simulink model "multitapdelay"  (Simulink 7.7)
settings: Solver=FixedStepDiscrete  StartTime=0.0  StopTime=10.0  RelTol=1e-3
libraries: dspsigops x2, dspsrcs4 x1, dspmtrx3 x1, dspsnks4 x1
settings Model: Creator=Arun  LastModifiedBy=Arun

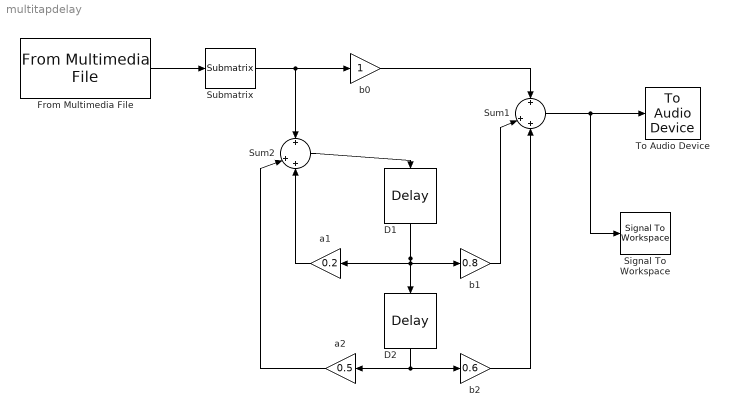
== system multitapdelay ==
  D1 : dspsigops/Delay  InputProcessing=Columns as channels (frame based)  dly_unit=Samples  delay=3000  ic_detail=off  dif_ic_for_ch=off  dif_ic_for_dly=off  ic=0  reset_popup=None
  D2 : dspsigops/Delay  InputProcessing=Columns as channels (frame based)  dly_unit=Samples  delay=1500  ic_detail=off  dif_ic_for_ch=off  dif_ic_for_dly=off  ic=0  reset_popup=None
  From Multimedia File : dspsrcs4/From Multimedia File  inputFilename=I:\Documents and Settings\Arun\Desktop\monayi\speech_dft.wav  loop=on  numPlays=1  outputStreams=Audio only  videoDataType=single  audioDataType=double  inheritSampleTime=on  userDefinedSampleTime=1/30  noAudioOutput=off  isIntensityVideo=off  fourcc=RGB  colorVideoFormat=Separate color signals  outputEOF=off  dataOrg=Column-major  audioFrameSize=1  computeAudioFrameSize=off
  Signal To Workspace : SignalToWorkspace  VariableName=audio_out  SaveFormat=Array  Save2DMode=2-D array (concatenate along first dimension)
      settings: CopyFcn=dspblkcopystw(gcbh);
  Submatrix : dspmtrx3/Submatrix  RowSpan=All rows  RowStartMode=First  RowStartIndex=1  RowEndMode=Last  RowEndIndex=1  ColSpan=One column  ColStartMode=First  ColStartIndex=1  ColEndMode=Last  ColEndIndex=1
  Sum1 : Sum  Inputs=+|++
  Sum2 : Sum  Inputs=+|++
  To Audio Device : dspsnks4/To Audio Device  deviceName=Default  inheritSampleRate=on  sampleRate=44100  deviceDatatype=Determine from input data type  autoBufferSize=on  bufferSize=4096  queueDuration=1.0
  a1 : Gain  Gain=0.2
  a2 : Gain  Gain=0.5
  b0 : Gain
  b1 : Gain  Gain=0.8
  b2 : Gain  Gain=0.6
  wires:
  From Multimedia File/1 -> Submatrix/1
  Submatrix/1 -> Sum2/1, b0/1
  b0/1 -> Sum1/1
  Sum1/1 -> To Audio Device/1, Signal To Workspace/1
  Sum2/1 -> D1/1
  b2/1 -> Sum1/3
  b1/1 -> Sum1/2
  a2/1 -> Sum2/2
  a1/1 -> Sum2/3
  D1/1 -> a1/1, b1/1, D2/1
  D2/1 -> a2/1, b2/1
